simulink model "Water_Pump"  (R2016b)
settings: Solver=FixedStepDiscrete  StartTime=0.0  StopTime=inf  FixedStep=WtrPmp.tiSimnTiStep_C.Value  RelTol=1e-3  EnableMultiTasking=on
settings Model: Creator=djuenema  LastModifiedBy=djuenema
settings DataIOCC: SaveFormat=StructureWithTime  SaveOutput=off  DSMLogging=off  VisualizeSimOutput=off  SaveTime=off  SignalLoggingName=Results
settings OptimizationCC: BlockReduction=off  ConditionallyExecuteInputs=off  LifeSpan=inf
settings DebuggingCC: AllowSymbolicDim=off  SFUnexpectedBacktrackingDiag=warning  SFNoUnconditionalDefaultTransitionDiag=warning  SFExecutionAtInitializationDiag=none
settings ModelReferenceCC: ModelReferenceNumInstancesAllowed=Single  PropagateSignalLabelsOutOfModel=off
settings GRTTargetCC: TargetLangStandard=C89/C90 (ANSI)
settings ConfigComp: CovMetricSettings=dw  CovHtmlReporting=on  CovSaveCumulativeToWorkspaceVar=on  CovSaveSingleToWorkspaceVar=on  CovExternalEMLEnable=off

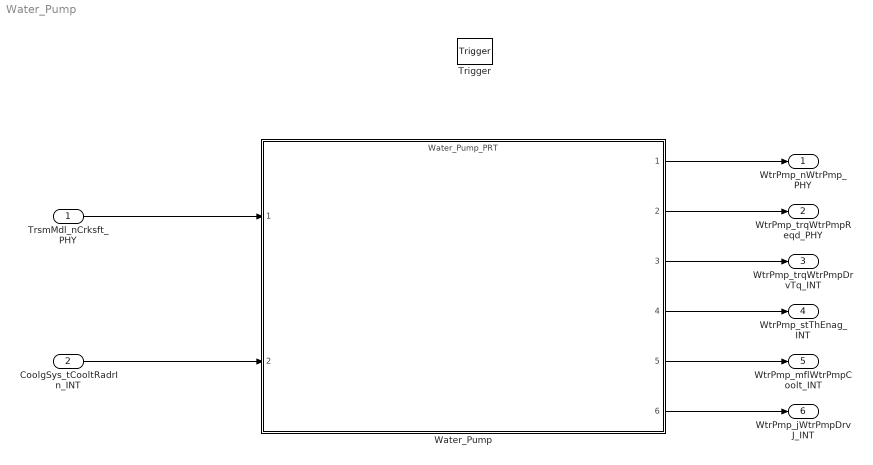
== system Water_Pump ==
  TrsmMdl_nCrksft_PHY : Inport
  CoolgSys_tCooltRadrIn_INT : Inport  Port=2
  Trigger : TriggerPort  TriggerType=function-call  VariantControl=Variant  PortDimensions=1
  Water_Pump : ModelReference  ModelNameDialog=Water_Pump_PRT.slxp  ModelReferenceVersion=1.3  CopyOfModelProtected=on
  WtrPmp_nWtrPmp_PHY : Outport
  WtrPmp_trqWtrPmpReqd_PHY : Outport  Port=2
  WtrPmp_trqWtrPmpDrvTq_INT : Outport  Port=3
  WtrPmp_stThEnag_INT : Outport  Port=4
  WtrPmp_mflWtrPmpCoolt_INT : Outport  Port=5
  WtrPmp_jWtrPmpDrvJ_INT : Outport  Port=6
  wires:
  Water_Pump/3 -> WtrPmp_trqWtrPmpDrvTq_INT/1
  Water_Pump/2 -> WtrPmp_trqWtrPmpReqd_PHY/1
  Water_Pump/1 -> WtrPmp_nWtrPmp_PHY/1
  Water_Pump/6 -> WtrPmp_jWtrPmpDrvJ_INT/1
  Water_Pump/4 -> WtrPmp_stThEnag_INT/1
  Water_Pump/5 -> WtrPmp_mflWtrPmpCoolt_INT/1
  CoolgSys_tCooltRadrIn_INT/1 -> Water_Pump/2
  TrsmMdl_nCrksft_PHY/1 -> Water_Pump/1
